simulink model "model1"  (R2020a)
settings: Solver=FixedStepAuto  StartTime=0.0  StopTime=20  FixedStep=0.001  RelTol=1e-3
undefined symbols (not defined in the file): w
libraries: simulink x1
settings Model: Creator=corte  LastModifiedBy=corte

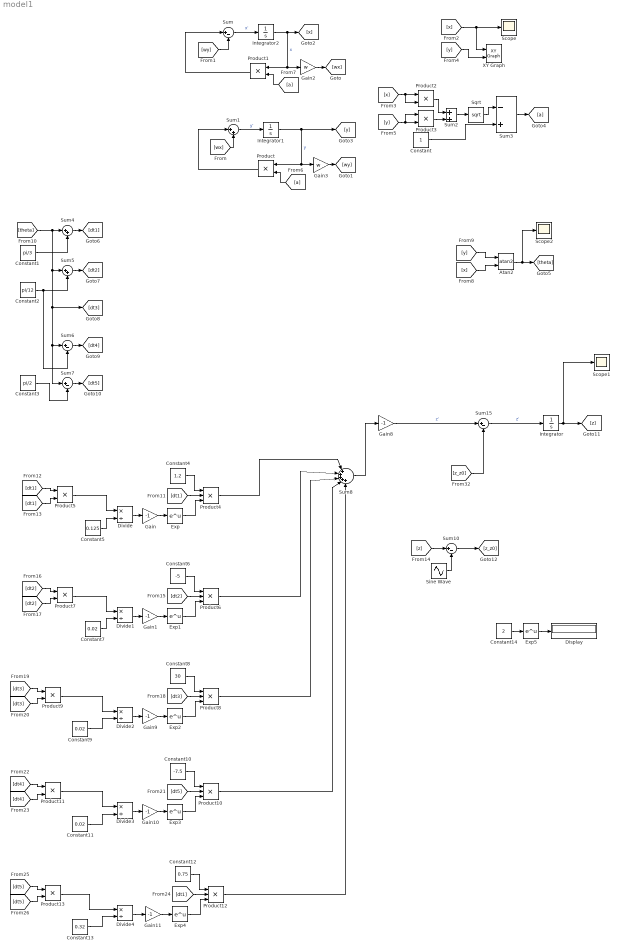
== system model1 ==
  Atan2 : Trigonometry  Operator=atan2
  Constant : Constant
  Constant1 : Constant  Value=pi/3
  Constant10 : Constant  Value=-7.5
  Constant11 : Constant  Value=0.02
  Constant12 : Constant  Value=0.75
  Constant13 : Constant  Value=0.32
  Constant14 : Constant  Value=2
  Constant2 : Constant  Value=pi/12
  Constant3 : Constant  Value=pi/2
  Constant4 : Constant  Value=1.2
  Constant5 : Constant  Value=0.125
  Constant6 : Constant  Value=-5
  Constant7 : Constant  Value=0.02
  Constant8 : Constant  Value=30
  Constant9 : Constant  Value=0.02
  Display : Display
  Divide{,1..4} (5 alike) : Product  Inputs=*/
  Exp{,1..5} (6 alike) : Math  SaturateOnIntegerOverflow=on
  Gain{,1,8..11} (6 alike) : Gain  Gain=-1
  Gain2 : Gain  Gain=w
  Gain3 : Gain  Gain=w
  Integrator : Integrator
  Integrator1 : Integrator
  Integrator2 : Integrator  InitialCondition=0.1
  Product{,1..3,5,7,9,11,13} (9 alike) : Product
  Product{4,6,8,10,12} (5 alike) : Product  Inputs=3
  Scope : Scope
  Scope1 : Scope
  Scope2 : Scope
  Sine Wave : Sin  Amplitude=0.15e-3  Frequency=pi/2  SampleTime=0
  Sqrt : Sqrt  SaturateOnIntegerOverflow=on
  Sum{,6..7,10,15} (5 alike) : Sum  Inputs=|+-
  Sum{1..2,4..5} (4 alike) : Sum  Inputs=|++
  Sum3 : Sum  Inputs=|-+
  Sum8 : Sum  Inputs=|+++++
  XY Graph : simulink/Sinks/XY Graph  xmin=-1.2  xmax=1.2  ymin=-1.2  ymax=1.2  st=-1
  wires:
  Sum/1 -> Integrator2/1  "x'"
  Integrator2/1 -> [x], Gain2/1, Product1/1  "x"
  Sum1/1 -> Integrator1/1  "y'"
  Integrator1/1 -> [y], Product/1, Gain3/1  "y"
  Gain2/1 -> [wx]
  [wx] -> Sum1/2
  Gain3/1 -> [wy]
  [wy] -> Sum/2
  [x] -> Scope/1, XY Graph/1
  Sum2/1 -> Sqrt/1
  [y] -> XY Graph/2
  Constant/1 -> Sum3/2
  Sqrt/1 -> Sum3/1
  Sum3/1 -> [a]
  [a] -> Product/2
  Product/1 -> Sum1/1
  Product1/1 -> Sum/1
  [a] -> Product1/2
  Product3/1 -> Sum2/2
  Product2/1 -> Sum2/1
  [y] -> Product3/1, Product3/2
  [x] -> Product2/2, Product2/1
  [y] -> Atan2/1
  [x] -> Atan2/2
  Atan2/1 -> Scope2/1, [theta]
  [theta] -> Sum7/1, Sum6/1, [dt3], Sum5/1, Sum4/1
  Constant1/1 -> Sum4/2
  Sum4/1 -> [dt1]
  Constant2/1 -> Sum6/2, Sum5/2
  Sum5/1 -> [dt2]
  Sum6/1 -> [dt4]
  Sum7/1 -> [dt5]
  Constant3/1 -> Sum7/2
  Constant4/1 -> Product4/1
  [dt1] -> Product4/2
  Exp/1 -> Product4/3
  Divide/1 -> Gain/1
  [dt1] -> Product5/1
  [dt1] -> Product5/2
  Product5/1 -> Divide/1
  Constant5/1 -> Divide/2
  Sum8/1 -> Gain8/1
  Sine Wave/1 -> Sum10/2
  [z] -> Sum10/1
  Sum10/1 -> [z_z0]
  Constant7/1 -> Divide1/2
  Product7/1 -> Divide1/1
  [dt2] -> Product7/2
  [dt2] -> Product7/1
  Divide1/1 -> Gain1/1
  Exp1/1 -> Product6/3
  [dt2] -> Product6/2
  Constant6/1 -> Product6/1
  Constant8/1 -> Product8/1
  [dt3] -> Product8/2
  Exp2/1 -> Product8/3
  Divide2/1 -> Gain9/1
  [dt3] -> Product9/1
  [dt3] -> Product9/2
  Product9/1 -> Divide2/1
  Constant9/1 -> Divide2/2
  Constant11/1 -> Divide3/2
  Product11/1 -> Divide3/1
  [dt4] -> Product11/2
  [dt4] -> Product11/1
  Divide3/1 -> Gain10/1
  Exp3/1 -> Product10/3
  [dt5] -> Product10/2
  Constant10/1 -> Product10/1
  Constant12/1 -> Product12/1
  [dt1] -> Product12/2
  Exp4/1 -> Product12/3
  Divide4/1 -> Gain11/1
  [dt5] -> Product13/1
  [dt5] -> Product13/2
  Product13/1 -> Divide4/1
  Constant13/1 -> Divide4/2
  Product6/1 -> Sum8/2
  Product8/1 -> Sum8/3
  Product10/1 -> Sum8/4
  Product12/1 -> Sum8/5
  Sum15/1 -> Integrator/1  "z'"
  Integrator/1 -> Scope1/1, [z]
  Product4/1 -> Sum8/1
  Constant14/1 -> Exp5/1
  Exp5/1 -> Display/1
  Gain/1 -> Exp/1
  Gain1/1 -> Exp1/1
  Gain9/1 -> Exp2/1
  Gain10/1 -> Exp3/1
  Gain11/1 -> Exp4/1
  [z_z0] -> Sum15/2
  Gain8/1 -> Sum15/1  "z'"
